simulink model "sceneElements"  (R2023b)
settings: Solver=VariableStepAuto  StartTime=0.0  StopTime=8  RelTol=1e-3
libraries: sim3dautolib x5, simulink x1, sim3dlib x1
settings Model: Creator=Hazem Abdelaziz  LastModifiedBy=Hazem Abdelaziz

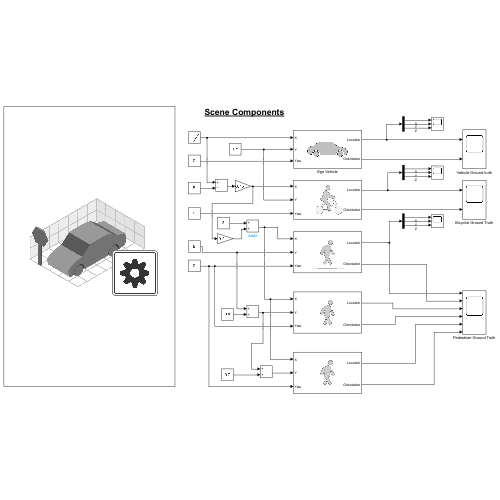
[thumbnail: Simulink's stored preview of the top-level diagram]
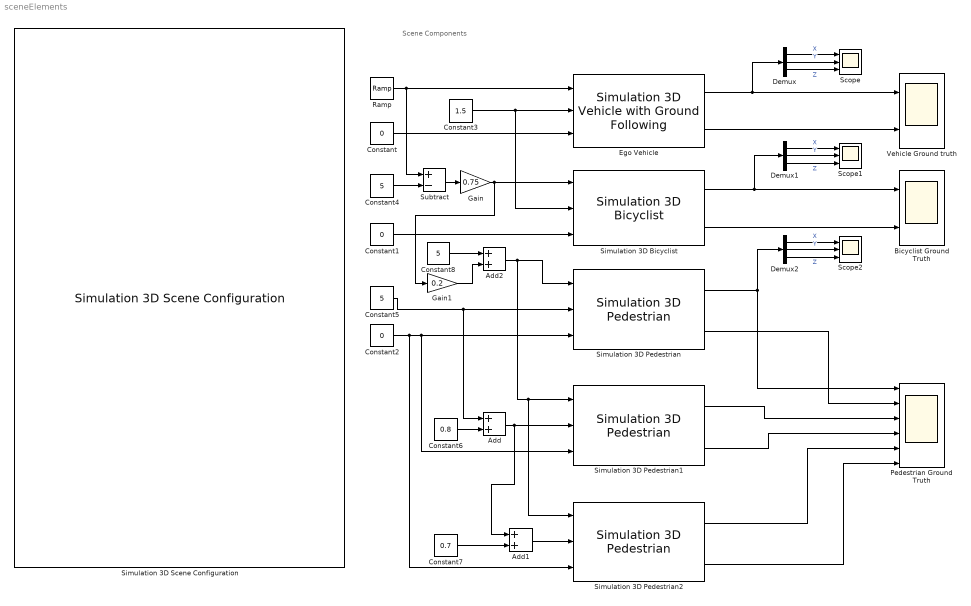
== system sceneElements ==
  note: Scene Components
  Add : Sum
  Add1 : Sum
  Add2 : Sum
  Bicyclist Ground Truth : Scope  NumInputPorts=2
  Constant : Constant  Value=0
  Constant1 : Constant  Value=0
  Constant2 : Constant  Value=0
  Constant3 : Constant  Value=1.5
  Constant4 : Constant  Value=5
  Constant5 : Constant  Value=5
  Constant6 : Constant  Value=0.8
  Constant7 : Constant  Value=0.7
  Constant8 : Constant  Value=5
  Demux : Demux  Outputs=3
  Demux1 : Demux  Outputs=3
  Demux2 : Demux  Outputs=3
  Ego Vehicle : sim3dautolib/Simulation 3D Vehicle with Ground Following  Priority=-1  PassVehMesh=Muscle car  MeshPath=/MathWorksAutomotiveContent/Vehicles/Muscle/Meshes/SK_MuscleCar.SK_MuscleCar  TrackWidth=1.9  WheelBase=3  WheelRadius=0.35  VehColor=Silver  InitialPos=[0, 0, 0]  InitialRot=[0, 0, 0]  ActorName=SimulinkVehicle1  SampleTime=-1  ActorType=SimulinkVehicle  ID=1  aMode=3  ActorTag=SimulinkVehicle1  CoordinateScheme=ISO  VehLightsControl=off  HeadlightColor=[ 1, 1, 1 ]  HighBeamIntensity=100000  LowBeamIntensity=60000  HighBeamConeAngle=70  LowBeamConeAngle=70  LeftHeadlightOrientation=[ 0, 0 ]  RightHeadlightOrientation=[ 0, 0 ]  BrakelightIntensity=500  ReverselightIntensity=500  SignallightIntensity=500  SignallightPeriod=1  SignalPulseWidth=50  TransformOutportEnabled=on
      settings: LibrarySourceBlock=drivingsim3d/Simulation 3D Vehicle with Ground Following
  Gain : Gain  Gain=0.75
  Gain1 : Gain  Gain=0.2
  Pedestrian Ground Truth : Scope  NumInputPorts=6
  Ramp : simulink/Sources/Ramp  slope=5  start=0  InitialOutput=0
  Scope : Scope  NumInputPorts=3
  Scope1 : Scope  NumInputPorts=3
  Scope2 : Scope  NumInputPorts=3
  Simulation 3D Bicyclist : sim3dautolib/Simulation 3D Bicyclist  Priority=-1  Scale=[1, 1, 1]  InitialPos=[0, 0, 0]  InitialRot=[0, 0, 0]  ActorName=SimulinkBicyclist1  SampleTime=-1  ActorType=SimulinkBicyclist  ActorTag=SimulinkBicyclist1  ID=1  aMode=3  CoordinateScheme=ISO  TransformOutportEnabled=on
      settings: LibrarySourceBlock=drivingsim3d/Simulation 3D Bicyclist
  Simulation 3D Pedestrian : sim3dautolib/Simulation 3D Pedestrian  Priority=-1  PedestrianType=Male 1  Scale=[1, 1, 1]  InitialPos=[0, 0, 0]  InitialYaw=0  ActorName=SimulinkPedestrian1  SampleTime=-1  ActorType=SimulinkPedestrian  ActorTag=SimulinkPedestrian1  ID=1  aMode=3  CoordinateScheme=ISO  TransformOutportEnabled=on
      settings: LibrarySourceBlock=drivingsim3d/Simulation 3D Pedestrian
  Simulation 3D Pedestrian1 : sim3dautolib/Simulation 3D Pedestrian  Priority=-1  PedestrianType=Female 2  Scale=[1, 1, 1]  InitialPos=[0, 0, 0]  InitialYaw=0  ActorName=SimulinkPedestrian2  SampleTime=-1  ActorType=SimulinkPedestrian  ActorTag=SimulinkPedestrian2  ID=2  aMode=3  CoordinateScheme=ISO  TransformOutportEnabled=on
      settings: LibrarySourceBlock=drivingsim3d/Simulation 3D Pedestrian
  Simulation 3D Pedestrian2 : sim3dautolib/Simulation 3D Pedestrian  Priority=-1  PedestrianType=Child  Scale=[1, 1, 1]  InitialPos=[0, 0, 0]  InitialYaw=0  ActorName=SimulinkPedestrian3  SampleTime=-1  ActorType=SimulinkPedestrian  ActorTag=SimulinkPedestrian3  ID=3  aMode=3  CoordinateScheme=ISO  TransformOutportEnabled=on
      settings: LibrarySourceBlock=drivingsim3d/Simulation 3D Pedestrian
  Simulation 3D Scene Configuration : sim3dlib/Simulation 3D Scene Configuration  Priority=0  ProjectFormat=Default Scenes  SceneDesc=US city block  ProjectName=C:\Program Files\MATLAB\R2023b\toolbox\shared\sim3d_projects\automotive_project_windows\UE\WindowsNoEditor\VehicleSimulation.exe  ScenePath=/Game/Maps/HwStrght  EnableOpenDRIVE=off  vehTagList={'Custom';'Scene Origin';'SimulinkVehicle1'}  vehTag=SimulinkVehicle1  FreeCameraInitialTranslation=[0, 0, 0]  FreeCameraDefaultInitialTranslation=[-6, 0, 2]  FreeCameraInitialRotation=[0, 0, 0]  FreeCameraDefaultInitialRotation=[0, -15, 0]  OpVisEn=off  Ts=1/60  EnableWindow=on  EnableRemoteAccess=off  EnableWeather=on  SunAltitude=25.200  SunAzimuth=90.0  clouds=10.0  wind=2.0  fog=5  rain=14.0  EnableGeospatial=off  OriginHeight=200  OriginLatitude=40.744652  OriginLongitude=-73.988864  MapStyle=Aerial  AdditionalAssetIDs=[]  UseAdvancedSunSky=off  SolarTime=11  TimeZone=-5  Day=21  Month=9  Year=2022  UseDaylightSavingTime=on  DSTStartDay=10  DSTStartMonth=3  DSTEndDay=3  DSTEndMonth=11  DSTSwitchHour=2  sensorTag=MainCamera1  sensorId=1  sensorName=MainCamera1  mountLoc=Origin  offsetFlag=off  tmountOffset=[0, 0, 0]  rmountOffset=[0, 0, 0]  HorizontalResolution=1280  VerticalResolution=720  HorizontalFOV=60  mountPoint=[0 0 0]  mountOrientation=[0 0 0]  aMode=3  ID=1  GeoTrigger=Inactive
      settings: LibrarySourceBlock=drivingsim3d/Simulation 3D Scene Configuration
  Subtract : Sum  Inputs=+-
  Vehicle Ground truth : Scope  NumInputPorts=2
  wires:
  Ego Vehicle/1 -> Demux/1, Vehicle Ground truth/1
  Ego Vehicle/2 -> Vehicle Ground truth/2
  Simulation 3D Bicyclist/2 -> Bicyclist Ground Truth/2
  Simulation 3D Pedestrian/2 -> Pedestrian Ground Truth/2
  Demux/1 -> Scope/1  "X"
  Demux/2 -> Scope/2  "Y"
  Demux/3 -> Scope/3  "Z"
  Gain/1 -> Simulation 3D Bicyclist/1, Gain1/1
  Demux1/3 -> Scope1/3  "Z"
  Simulation 3D Bicyclist/1 -> Demux1/1, Bicyclist Ground Truth/1
  Demux1/1 -> Scope1/1  "X"
  Demux1/2 -> Scope1/2  "Y"
  Constant/1 -> Ego Vehicle/3
  Constant1/1 -> Simulation 3D Bicyclist/3
  Constant2/1 -> Simulation 3D Pedestrian2/3, Simulation 3D Pedestrian1/3, Simulation 3D Pedestrian/3
  Simulation 3D Pedestrian/1 -> Demux2/1, Pedestrian Ground Truth/1
  Demux2/1 -> Scope2/1  "X"
  Demux2/3 -> Scope2/3  "Z"
  Demux2/2 -> Scope2/2  "Y"
  Gain1/1 -> Add2/2
  Ramp/1 -> Subtract/1, Ego Vehicle/1
  Constant3/1 -> Simulation 3D Bicyclist/2, Ego Vehicle/2
  Subtract/1 -> Gain/1
  Constant4/1 -> Subtract/2
  Constant5/1 -> Simulation 3D Pedestrian/2, Add/1
  Add/1 -> Simulation 3D Pedestrian1/2, Add1/1
  Constant6/1 -> Add/2
  Constant7/1 -> Add1/2
  Add1/1 -> Simulation 3D Pedestrian2/2
  Simulation 3D Pedestrian1/1 -> Pedestrian Ground Truth/3
  Simulation 3D Pedestrian1/2 -> Pedestrian Ground Truth/4
  Simulation 3D Pedestrian2/1 -> Pedestrian Ground Truth/5
  Simulation 3D Pedestrian2/2 -> Pedestrian Ground Truth/6
  Add2/1 -> Simulation 3D Pedestrian2/1, Simulation 3D Pedestrian1/1, Simulation 3D Pedestrian/1
  Constant8/1 -> Add2/1
